simulink model "sl_robot_sincrono_control"  (R2016b)
settings: Solver=VariableStepAuto  StartTime=0.0  StopTime=10  RelTol=1e-3
values from neighbouring files (symbols this model uses):
  omega_sat = [-0.2618 0.2618]    [prueba_persecucionPURA.m]    (also in pruebas_MCD.m; pruebas_MCI.m; pruebas_control.m; pruebas_control_P2.m)
  pos_init = [0;0;0]    [prueba_persecucionPURA.m]    (also in pruebas_MCD.m; pruebas_MCI.m; pruebas_control.m; pruebas_control_P2.m)
  tetha_d_sat = [-0.75 0.75]    [prueba_persecucionPURA.m]    (also in pruebas_MCD.m; pruebas_MCI.m; pruebas_control.m; pruebas_control_P2.m)
settings Model: Creator=marrcogrova  LastModifiedBy=marrcogrova

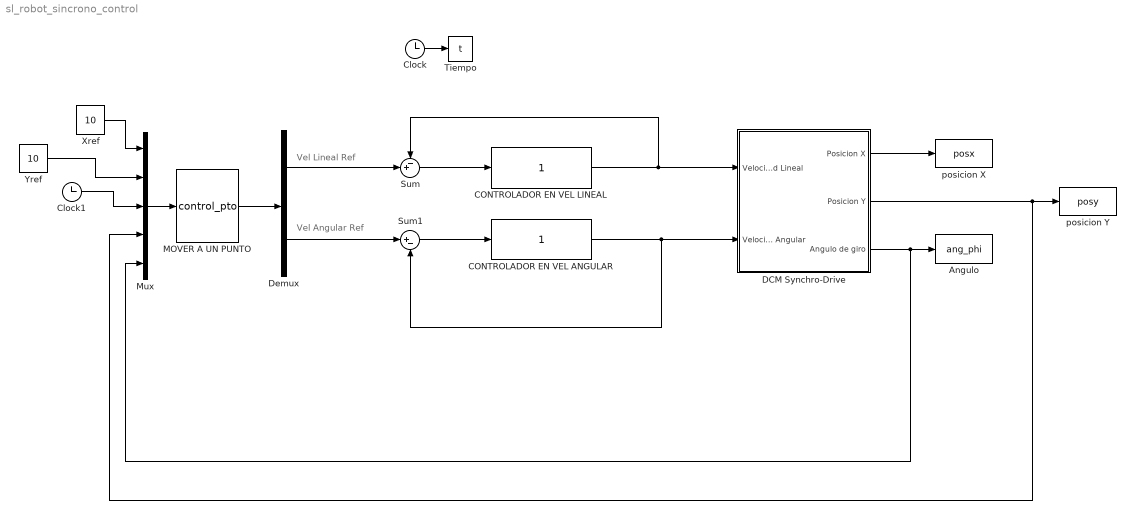
== system sl_robot_sincrono_control ==
  note: Vel Lineal Ref
  note: Vel Angular Ref
  Angulo : ToWorkspace  VariableName=ang_phi  SampleTime=-1
  CONTROLADOR EN VEL ANGULAR : MATLABFcn  MATLABFcn=1  OutputDimensions=1
  CONTROLADOR EN VEL LINEAL : MATLABFcn  MATLABFcn=1  OutputDimensions=1
  Clock : Clock
  Clock1 : Clock
  DCM Synchro-Drive : Subsystem
  Demux : Demux  Outputs=2
  MOVER A UN PUNTO : MATLABFcn  MATLABFcn=control_pto  OutputDimensions=2
  Mux : Mux  Inputs=5
  Sum : Sum  Inputs=-+|
  Sum1 : Sum  Inputs=|+-
  Tiempo : ToWorkspace  VariableName=t  SampleTime=-1
  Xref : Constant  Value=10
  Yref : Constant  Value=10
  posicion X : ToWorkspace  VariableName=posx  SampleTime=-1
  posicion Y : ToWorkspace  VariableName=posy  SampleTime=-1
  wires:
  Clock/1 -> Tiempo/1
  DCM Synchro-Drive/1(Posicion X) -> posicion X/1
  DCM Synchro-Drive/2(Posicion Y) -> Mux/4, posicion Y/1
  MOVER A UN PUNTO/1 -> Demux/1
  Mux/1 -> MOVER A UN PUNTO/1
  Xref/1 -> Mux/1
  Yref/1 -> Mux/2
  Clock1/1 -> Mux/3
  DCM Synchro-Drive/3(Angulo de giro) -> Mux/5, Angulo/1
  Demux/1 -> Sum/2
  Sum/1 -> CONTROLADOR EN VEL LINEAL/1
  Demux/2 -> Sum1/1
  Sum1/1 -> CONTROLADOR EN VEL ANGULAR/1
  CONTROLADOR EN VEL ANGULAR/1 -> DCM Synchro-Drive/2(Velocidad Angular), Sum1/2
  CONTROLADOR EN VEL LINEAL/1 -> Sum/1, DCM Synchro-Drive/1(Velocidad Lineal)

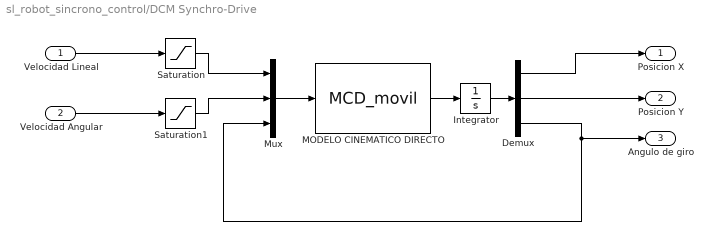
== system sl_robot_sincrono_control/DCM Synchro-Drive ==
  Velocidad Lineal : Inport
  Velocidad Angular : Inport  Port=2
  Demux : Demux  Outputs=3
  Integrator : Integrator  InitialCondition=pos_init
  MODELO CINEMATICO DIRECTO : MATLABFcn  MATLABFcn=MCD_movil  OutputDimensions=3
  Mux : Mux  Inputs=3
  Saturation : Saturate  UpperLimit=tetha_d_sat(2)  LowerLimit=tetha_d_sat(1)
  Saturation1 : Saturate  UpperLimit=omega_sat(2)  LowerLimit=omega_sat(1)
  Posicion X : Outport
  Posicion Y : Outport  Port=2
  Angulo de giro : Outport  Port=3
  wires:
  Integrator/1 -> Demux/1
  Demux/3 -> Angulo de giro/1, Mux/3
  Demux/1 -> Posicion X/1
  Demux/2 -> Posicion Y/1
  Mux/1 -> MODELO CINEMATICO DIRECTO/1
  MODELO CINEMATICO DIRECTO/1 -> Integrator/1
  Velocidad Lineal/1 -> Saturation/1
  Saturation/1 -> Mux/1
  Saturation1/1 -> Mux/2
  Velocidad Angular/1 -> Saturation1/1
